simulink model "Quadrotor_Model"  (R2025a)
settings: Solver=ode45  StartTime=0.0  StopTime=370  RelTol=1e-3  EnableMultiTasking=on
values from neighbouring files (symbols this model uses):
  b = 0.07    [project_launch.m]
  drone_mass = 2    [project_launch.m]
  g = 9.81    [project_launch.m]
  Ixx = 0.0231693085    [project_launch.m]
  Iyy = 0.0231693085    [project_launch.m]
  Izz = 0.0449757165    [project_launch.m]
  Jr = 6.8145025e-06    [project_launch.m]
  k = 0.09    [project_launch.m]
  K_d_phi = 0.0002    [project_launch.m]
  K_d_psi = 0.07    [project_launch.m]
  K_d_theta = 0.001    [project_launch.m]
  K_dx = 0.035    [project_launch.m]
  K_dy = 0.06    [project_launch.m]
  K_dz = 5    [project_launch.m]
  K_p_phi = 0.1    [project_launch.m]
  K_p_psi = 0.05    [project_launch.m]
  K_p_theta = 0.75    [project_launch.m]
  K_px = 0.6    [project_launch.m]
  K_py = 0.81    [project_launch.m]
  K_pz = 7    [project_launch.m]
  L = 0.1651    [project_launch.m]
  m = 2    [project_launch.m]
  w = 20    [project_launch.m]
settings Model: Creator=boyan  LastModifiedBy=Happy
settings SolverCC: MaxConsecutiveMinStep=2  AlgebraicLoopSolver=TrustRegion
settings DataIOCC: LimitDataPoints=on  SaveFormat=Array  ReturnWorkspaceOutputs=off
settings OptimizationCC: LifeSpan=inf
settings DebuggingCC: SolverPrmCheckMsg=warning  UnconnectedInputMsg=warning  UnconnectedOutputMsg=warning  UnconnectedLineMsg=warning  SFUnexpectedBacktrackingDiag=warning  SFNoUnconditionalDefaultTransitionDiag=warning  SFExecutionAtInitializationDiag=none  ArithmeticOperatorsInVariantConditions=warning
settings HardwareCC: ProdBitPerPointer=32.0  ProdBitPerSizeT=32.0  ProdBitPerPtrDiffT=32.0  ProdLargestAtomicFloat=None  ProdIntDivRoundTo=Undefined  ProdEndianess=Unspecified  ProdWordSize=32.0  ProdHWDeviceType=32-bit Generic
settings ModelReferenceCC: EnableRefExpFcnMdlSchedulingChecks=on  PropagateSignalLabelsOutOfModel=off
settings SFSimCC: SimUseLocalCustomCode=off  CustomCodeUndefinedFunction=UseInterfaceOnly
settings RTWCC: RTWUseLocalCustomCode=off  GPUComputeCapability=3.5  DLArmComputeVersion=19.05
settings CodeAppCC: StateflowObjectComments=on
settings GRTTargetCC: TargetLangStandard=C89/C90 (ANSI)
settings ConfigComp: CovMetricSettings=dw  CovSaveCumulativeToWorkspaceVar=on  CovSaveSingleToWorkspaceVar=on  CovExternalEMLEnable=off  CovSFcnEnable=off

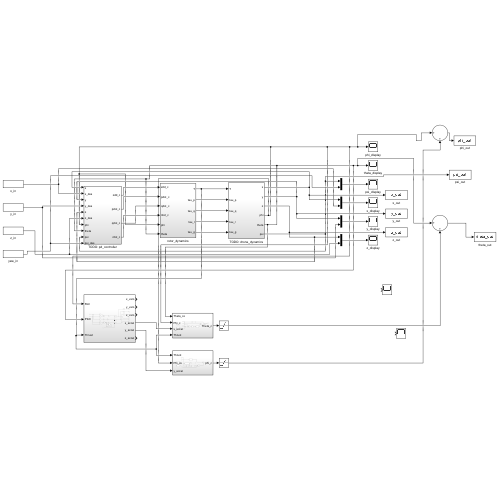
[thumbnail: Simulink's stored preview of the top-level diagram]
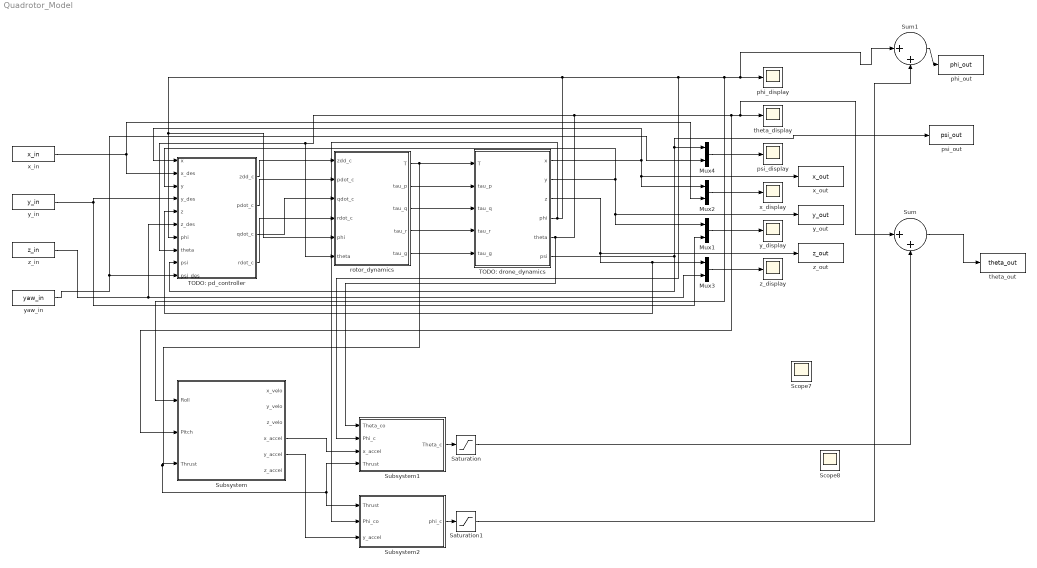
== system Quadrotor_Model ==
  Mux{1..4} (4 alike) : Mux  Inputs=2
  Saturation : Saturate  UpperLimit=160  LowerLimit=-160
  Saturation1 : Saturate  UpperLimit=160  LowerLimit=-160
  Scope7 : Scope
      settings: ActiveDisplayYMinimum=-1.6883197970171271  ActiveDisplayYMaximum=2.5090035346084125  DataLoggingVariableName=ScopeData12
  Scope8 : Scope
      settings: ActiveDisplayYMinimum=-0.67404865904457345  ActiveDisplayYMaximum=1.0700258804030376  DataLoggingVariableName=ScopeData10
  Subsystem : Subsystem
  Subsystem1 : Subsystem
  Subsystem2 : Subsystem
  Sum : Sum  Inputs=|++
  Sum1 : Sum  Inputs=|++
  TODO: drone_dynamics : Subsystem
  TODO: pd_controller : Subsystem
  phi_display : Scope
      settings: ActiveDisplayYMinimum=-3.14  ActiveDisplayYMaximum=3.14
  phi_out : ToWorkspace  VariableName=phi_out  SaveFormat=Timeseries  SampleTime=-1
  psi_display : Scope
      settings: ActiveDisplayYMinimum=-0.78539816339744806  ActiveDisplayYMaximum=7.0685834705770345  DataLoggingVariableName=ScopeData2
  psi_out : ToWorkspace  VariableName=psi_out  SaveFormat=Timeseries  SampleTime=-1
  rotor_dynamics : Subsystem
  theta_display : Scope
      settings: ActiveDisplayYMinimum=-3.14  ActiveDisplayYMaximum=3.14  DataLoggingVariableName=ScopeData3
  theta_out : ToWorkspace  VariableName=theta_out  SaveFormat=Timeseries  SampleTime=-1
  x_display : Scope
      settings: ActiveDisplayYMinimum=-200  DataLoggingVariableName=ScopeData4
  x_in : FromWorkspace  VariableName=x_in
  x_out : ToWorkspace  VariableName=x_out  SaveFormat=Timeseries  SampleTime=-1
  y_display : Scope
      settings: ActiveDisplayYMinimum=-20  ActiveDisplayYMaximum=140  DataLoggingVariableName=ScopeData5
  y_in : FromWorkspace  VariableName=y_in
  y_out : ToWorkspace  VariableName=y_out  SaveFormat=Timeseries  SampleTime=-1
  yaw_in : FromWorkspace  VariableName=yaw_in
  z_display : Scope
      settings: ActiveDisplayYMinimum=-50
  z_in : FromWorkspace  VariableName=z_in
  z_out : ToWorkspace  VariableName=z_out  SaveFormat=Timeseries  SampleTime=-1
  wires:
  rotor_dynamics/2(tau_p) -> TODO: drone_dynamics/2(tau_p)
  TODO: pd_controller/1(zdd_c) -> rotor_dynamics/1(zdd_c)
  TODO: pd_controller/2(pdot_c) -> rotor_dynamics/2(pdot_c)
  z_in/1 -> TODO: pd_controller/6(z_des), Mux3/2
  Mux1/1 -> y_display/1
  Mux2/1 -> x_display/1
  Mux4/1 -> psi_display/1
  Mux3/1 -> z_display/1
  TODO: drone_dynamics/6(psi) -> TODO: pd_controller/9(psi), psi_out/1, Mux4/1
  y_in/1 -> Mux1/2, TODO: pd_controller/4(y_des)
  x_in/1 -> Mux2/2, TODO: pd_controller/2(x_des)
  TODO: drone_dynamics/3(z) -> z_out/1, TODO: pd_controller/5(z), Mux3/1
  TODO: drone_dynamics/5(theta) -> Subsystem1/1(Theta_co), Subsystem/2(Pitch), Sum/1, theta_display/1, rotor_dynamics/6(theta), TODO: pd_controller/8(theta)
  TODO: drone_dynamics/2(y) -> Mux1/1, y_out/1, TODO: pd_controller/3(y)
  TODO: drone_dynamics/4(phi) -> Subsystem2/2(Phi_co), Subsystem1/2(Phi_c), Subsystem/1(Roll), Sum1/1, phi_display/1, rotor_dynamics/5(phi), TODO: pd_controller/7(phi)
  TODO: drone_dynamics/1(x) -> Mux2/1, x_out/1, TODO: pd_controller/1(x)
  rotor_dynamics/5(tau_g) -> TODO: drone_dynamics/5(tau_g)
  rotor_dynamics/3(tau_q) -> TODO: drone_dynamics/3(tau_q)
  rotor_dynamics/4(tau_r) -> TODO: drone_dynamics/4(tau_r)
  yaw_in/1 -> Mux4/2, TODO: pd_controller/10(psi_des)
  TODO: pd_controller/4(rdot_c) -> rotor_dynamics/4(rdot_c)
  TODO: pd_controller/3(qdot_c) -> rotor_dynamics/3(qdot_c)
  rotor_dynamics/1(T) -> Subsystem/3(Thrust), Subsystem1/4(Thrust), Subsystem2/1(Thrust), TODO: drone_dynamics/1(T)
  Saturation1/1 -> Sum1/2
  Subsystem/5(y_accel) -> Subsystem2/3(y_accel)
  Subsystem2/1(phi_c) -> Saturation1/1
  Subsystem1/1(Theta_c) -> Saturation/1
  Subsystem/4(x_accel) -> Subsystem1/3(x_accel)
  Sum/1 -> theta_out/1
  Saturation/1 -> Sum/2
  Sum1/1 -> phi_out/1

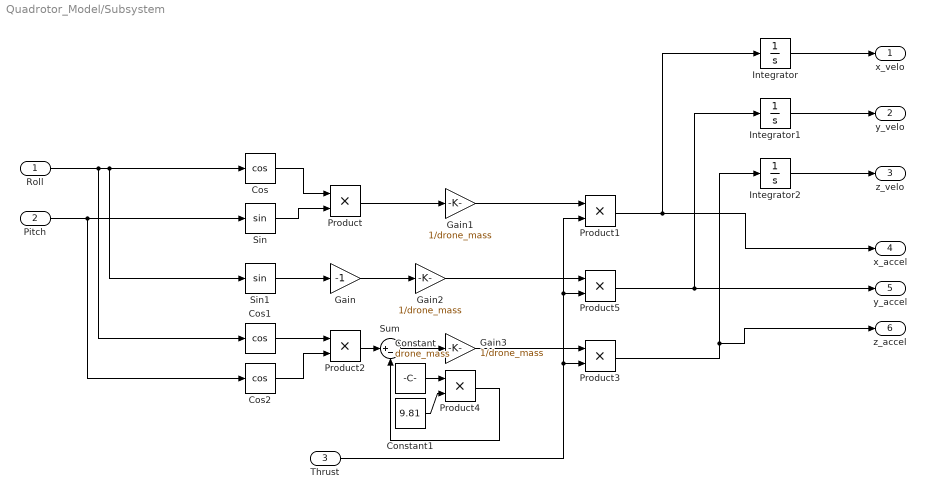
== system Quadrotor_Model/Subsystem ==
  Roll : Inport
  Pitch : Inport  Port=2
  Thrust : Inport  Port=3
  Constant : Constant  Value=drone_mass
  Constant1 : Constant  Value=9.81
  Cos : Trigonometry  Operator=cos
  Cos1 : Trigonometry  Operator=cos
  Cos2 : Trigonometry  Operator=cos
  Gain : Gain  Gain=-1
  Gain1 : Gain  Gain=1/drone_mass
  Gain2 : Gain  Gain=1/drone_mass
  Gain3 : Gain  Gain=1/drone_mass
  Integrator : Integrator
  Integrator1 : Integrator
  Integrator2 : Integrator
  Product{,1..5} (6 alike) : Product
  Sin : Trigonometry
  Sin1 : Trigonometry
  Sum : Sum  Inputs=|+-
  x_velo : Outport
  y_velo : Outport  Port=2
  z_velo : Outport  Port=3
  x_accel : Outport  Port=4
  y_accel : Outport  Port=5
  z_accel : Outport  Port=6
  wires:
  Sin/1 -> Product/2
  Cos/1 -> Product/1
  Pitch/1 -> Sin/1, Cos2/1
  Roll/1 -> Cos1/1, Cos/1, Sin1/1
  Sin1/1 -> Gain/1
  Cos2/1 -> Product2/2
  Cos1/1 -> Product2/1
  Constant/1 -> Product4/1
  Constant1/1 -> Product4/2
  Product4/1 -> Sum/2
  Sum/1 -> Gain3/1
  Thrust/1 -> Product1/2, Product5/2, Product3/2
  Gain/1 -> Gain2/1
  Product/1 -> Gain1/1
  Gain1/1 -> Product1/1
  Gain2/1 -> Product5/1
  Product2/1 -> Sum/1
  Product5/1 -> Integrator1/1, y_accel/1
  Product3/1 -> Integrator2/1, z_accel/1
  Integrator2/1 -> z_velo/1
  Integrator1/1 -> y_velo/1
  Integrator/1 -> x_velo/1
  Product1/1 -> Integrator/1, x_accel/1
  Gain3/1 -> Product3/1

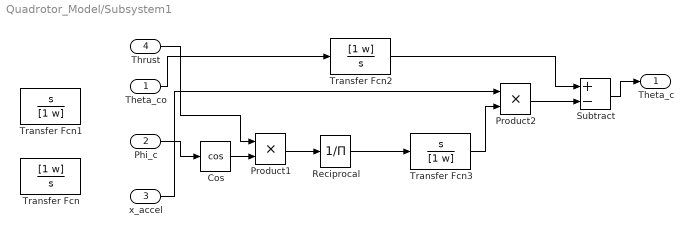
== system Quadrotor_Model/Subsystem1 ==
  Theta_co : Inport
  Phi_c : Inport  Port=2
  x_accel : Inport  Port=3
  Thrust : Inport  Port=4
  Cos : Trigonometry  Operator=cos
  Product1 : Product
  Product2 : Product
  Reciprocal : Product  Inputs=/
  Subtract : Sum  Inputs=+-
  Transfer Fcn : TransferFcn  Numerator=[1 w]  Denominator=[1 0]
  Transfer Fcn1 : TransferFcn  Numerator=[1 0]  Denominator=[1 w]
  Transfer Fcn2 : TransferFcn  Numerator=[1 w]  Denominator=[1 0]
  Transfer Fcn3 : TransferFcn  Numerator=[1 0]  Denominator=[1 w]
  Theta_c : Outport
  wires:
  Theta_co/1 -> Transfer Fcn2/1
  Cos/1 -> Product1/2
  Phi_c/1 -> Cos/1
  Product1/1 -> Reciprocal/1
  x_accel/1 -> Product2/1
  Product2/1 -> Subtract/2
  Transfer Fcn2/1 -> Subtract/1
  Subtract/1 -> Theta_c/1
  Thrust/1 -> Product1/1
  Reciprocal/1 -> Transfer Fcn3/1
  Transfer Fcn3/1 -> Product2/2

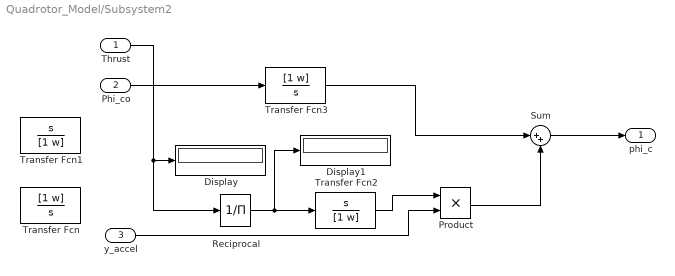
== system Quadrotor_Model/Subsystem2 ==
  Thrust : Inport
  Phi_co : Inport  Port=2
  y_accel : Inport  Port=3
  Display : Display
  Display1 : Display
  Product : Product
  Reciprocal : Product  Inputs=/
  Sum : Sum  Inputs=|++
  Transfer Fcn : TransferFcn  Numerator=[1 w]  Denominator=[1 0]
  Transfer Fcn1 : TransferFcn  Numerator=[1 0]  Denominator=[1 w]
  Transfer Fcn2 : TransferFcn  Numerator=[1 0]  Denominator=[1 w]
  Transfer Fcn3 : TransferFcn  Numerator=[1 w]  Denominator=[1 0]
  phi_c : Outport
  wires:
  Reciprocal/1 -> Display1/1, Transfer Fcn2/1
  y_accel/1 -> Product/2
  Transfer Fcn2/1 -> Product/1
  Product/1 -> Sum/2
  Phi_co/1 -> Transfer Fcn3/1
  Transfer Fcn3/1 -> Sum/1
  Sum/1 -> phi_c/1
  Thrust/1 -> Display/1, Reciprocal/1

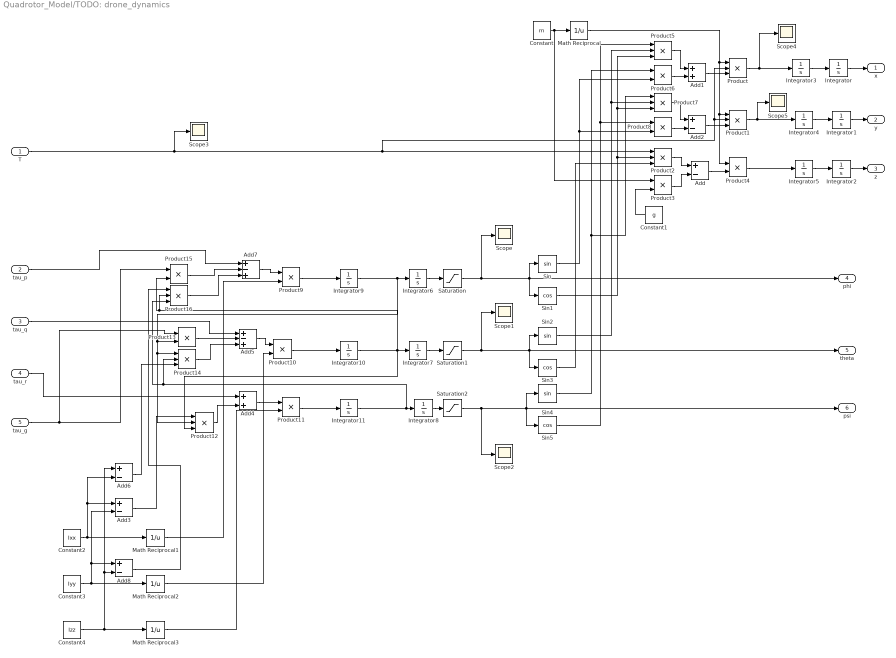
== system Quadrotor_Model/TODO: drone_dynamics ==
  T : Inport
  tau_p : Inport  Port=2
  tau_q : Inport  Port=3
  tau_r : Inport  Port=4
  tau_g : Inport  Port=5
  Add{,2..3,6,8} (5 alike) : Sum  Inputs=+-
  Add1 : Sum
  Add4 : Sum
  Add5 : Sum  Inputs=+-+
  Add7 : Sum  Inputs=+-+
  Constant : Constant  Value=m
  Constant1 : Constant  Value=g
  Constant2 : Constant  Value=Ixx
  Constant3 : Constant  Value=Iyy
  Constant4 : Constant  Value=Izz
  Integrator{,1..7,9..11} (11 alike) : Integrator
  Integrator8 : Integrator  WrappedStateUpperValue=2*pi  WrappedStateLowerValue=0
  Math Reciprocal{,1..3} (4 alike) : Math  Operator=reciprocal  SignedPower=on
  Product{,1..2,5,7,12,14,16} (8 alike) : Product  Inputs=3
  Product{3..4,6,8..11,13,15} (9 alike) : Product
  Saturation : Saturate  UpperLimit=1  LowerLimit=-1
  Saturation1 : Saturate  UpperLimit=1  LowerLimit=-1
  Saturation2 : Saturate  UpperLimit=2*pi  LowerLimit=0
  Scope{,1..5} (6 alike) : Scope
      Scope settings: ActiveDisplayYMinimum=-3.15  ActiveDisplayYMaximum=3.15
      Scope1 settings: ActiveDisplayYMinimum=-4.8E-9  ActiveDisplayYMaximum=6E-10  DataLoggingVariableName=ScopeData2
      Scope2 settings: ActiveDisplayYMinimum=-0.8979  ActiveDisplayYMaximum=7.08108  DataLoggingVariableName=ScopeData3
      Scope3 settings: ActiveDisplayYMinimum=-3.4849041226239738E+14  ActiveDisplayYMaximum=4.4753425626299984E+13  DataLoggingVariableName=ScopeData4
      Scope4 settings: ActiveDisplayYMinimum=-1.5375275296905083E+12  ActiveDisplayYMaximum=8.56477193990877E+11  DataLoggingVariableName=ScopeData5
      Scope5 settings: DataLoggingVariableName=ScopeData6
  Sin : Trigonometry
  Sin1 : Trigonometry  Operator=cos
  Sin2 : Trigonometry
  Sin3 : Trigonometry  Operator=cos
  Sin4 : Trigonometry
  Sin5 : Trigonometry  Operator=cos
  x : Outport
  y : Outport  Port=2
  z : Outport  Port=3
  phi : Outport  Port=4
  theta : Outport  Port=5
  psi : Outport  Port=6
  wires:
  Math Reciprocal1/1 -> Product9/2
  Add5/1 -> Product10/1
  Add7/1 -> Product9/1
  Product9/1 -> Integrator9/1
  Add/1 -> Product4/2
  Product4/1 -> Integrator5/1
  Sin1/1 -> Product2/2, Product7/3, Product5/3
  Constant2/1 -> Math Reciprocal1/1, Add6/2, Add3/1
  Integrator11/1 -> Product16/3, Product14/2, Integrator8/1
  Integrator/1 -> x/1
  Sin/1 -> Product8/2, Product6/2
  Sin3/1 -> Product2/3
  T/1 -> Scope3/1, Product/2, Product1/2, Product2/1
  Constant4/1 -> Math Reciprocal3/1, Add8/2, Add6/1
  Add6/1 -> Product14/3
  Integrator4/1 -> Integrator1/1
  Product5/1 -> Add1/1
  Math Reciprocal3/1 -> Product11/2
  Product11/1 -> Integrator11/1
  Integrator6/1 -> Saturation/1
  Integrator9/1 -> Product12/2, Product14/1, Product13/2, Integrator6/1
  Product6/1 -> Add1/2
  Product14/1 -> Add5/3
  Add8/1 -> Product16/1
  Integrator5/1 -> Integrator2/1
  Constant1/1 -> Product3/2
  Product16/1 -> Add7/3
  Saturation2/1 -> psi/1, Sin5/1, Sin4/1, Scope2/1
  Add1/1 -> Product/3
  Integrator3/1 -> Integrator/1
  Saturation/1 -> phi/1, Sin1/1, Sin/1, Scope/1
  Integrator7/1 -> Saturation1/1
  Sin5/1 -> Product8/1, Product5/1
  tau_p/1 -> Add7/1
  Sin4/1 -> Product7/1, Product6/1
  Constant3/1 -> Add8/1, Add3/2, Math Reciprocal2/1
  Add3/1 -> Product12/1
  Product7/1 -> Add2/1
  Math Reciprocal2/1 -> Product10/2
  Product13/1 -> Add5/2
  Integrator1/1 -> y/1
  Product2/1 -> Add/1
  Add2/1 -> Product1/3
  Product15/1 -> Add7/2
  tau_g/1 -> Product15/1, Product13/1
  Product10/1 -> Integrator10/1
  Sin2/1 -> Product5/2, Product7/2
  Product/1 -> Scope4/1, Integrator3/1
  Product8/1 -> Add2/2
  Math Reciprocal/1 -> Product/1, Product4/1, Product1/1
  Integrator2/1 -> z/1
  Product12/1 -> Add4/2
  Product3/1 -> Add/2
  tau_r/1 -> Add4/1
  Product1/1 -> Scope5/1, Integrator4/1
  Constant/1 -> Math Reciprocal/1, Product3/1
  Saturation1/1 -> Sin3/1, theta/1, Sin2/1, Scope1/1
  Add4/1 -> Product11/1
  Integrator8/1 -> Saturation2/1
  Integrator10/1 -> Product12/3, Product16/2, Product15/2, Integrator7/1
  tau_q/1 -> Add5/1

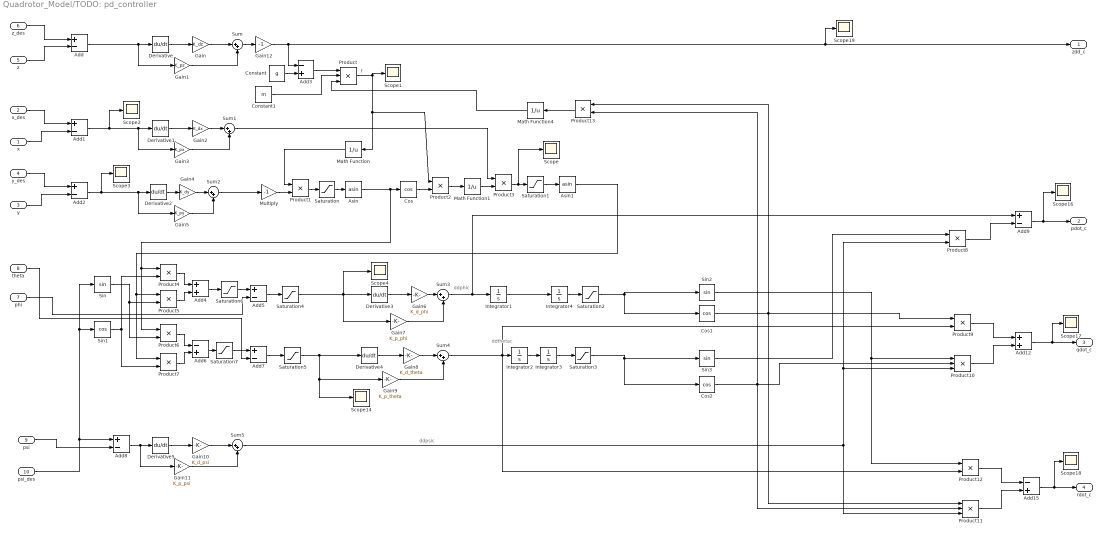
== system Quadrotor_Model/TODO: pd_controller ==
  note: ddphic
  note: ddthetac
  note: f
  note: ddpsic
  x : Inport
  x_des : Inport  Port=2
  y : Inport  Port=3
  y_des : Inport  Port=4
  z : Inport  Port=5
  z_des : Inport  Port=6
  phi : Inport  Port=7
  theta : Inport  Port=8
  psi : Inport  Port=9
  psi_des : Inport  Port=10
  Add{,1..2,5,7..9} (7 alike) : Sum  Inputs=+-
  Add12 : Sum
  Add15 : Sum  Inputs=-+
  Add3 : Sum  Inputs=-+
  Add4 : Sum
  Add6 : Sum  Inputs=-+
  Asin : Trigonometry  Operator=asin
  Asin1 : Trigonometry  Operator=asin
  Constant : Constant  Value=g
  Constant1 : Constant  Value=m
  Cos : Trigonometry  Operator=cos
  Cos1 : Trigonometry  Operator=cos
  Cos2 : Trigonometry  Operator=cos
  Derivative{,1..5} (6 alike) : Derivative
  Gain : Gain  Gain=K_dz
  Gain1 : Gain  Gain=K_pz
  Gain10 : Gain  Gain=K_d_psi
  Gain11 : Gain  Gain=K_p_psi
  Gain12 : Gain  Gain=-1
  Gain2 : Gain  Gain=K_dx
  Gain3 : Gain  Gain=K_px
  Gain4 : Gain  Gain=K_dy
  Gain5 : Gain  Gain=K_py
  Gain6 : Gain  Gain=K_d_phi
  Gain7 : Gain  Gain=K_p_phi
  Gain8 : Gain  Gain=K_d_theta
  Gain9 : Gain  Gain=K_p_theta
  Integrator{1..4} (4 alike) : Integrator
  Math Function : Math  Operator=reciprocal
  Math Function1 : Math  Operator=reciprocal
  Math Function4 : Math  Operator=reciprocal
  Multiply : Gain  Gain=-1
  Product : Product  Inputs=3
  Product{1..9,12..13} (11 alike) : Product
  Product10 : Product  Inputs=3
  Product11 : Product  Inputs=3
  Saturation{,1..3,6..7} (6 alike) : Saturate  UpperLimit=1  LowerLimit=-1  ZeroCross=off
  Saturation4 : Saturate  UpperLimit=0.2  LowerLimit=-0.2  ZeroCross=off
  Saturation5 : Saturate  UpperLimit=0.1  LowerLimit=-0.1  ZeroCross=off
  Scope{,1..4,14,16..19} (10 alike) : Scope
      Scope settings: ActiveDisplayYMinimum=-3E-11  ActiveDisplayYMaximum=2E-10  DataLoggingVariableName=ScopeData7
      Scope1 settings: ActiveDisplayYMinimum=-4.3522364874412031E+14  ActiveDisplayYMaximum=5.24366948093118E+13
      Scope14 settings: ActiveDisplayYMinimum=-2.2  ActiveDisplayYMaximum=2.2  DataLoggingVariableName=ScopeData13
      Scope16 settings: ActiveDisplayYMinimum=-0.00891  ActiveDisplayYMaximum=0.00408  DataLoggingVariableName=ScopeData15
      Scope17 settings: ActiveDisplayYMinimum=-0.01  ActiveDisplayYMaximum=0.01  DataLoggingVariableName=ScopeData16
      Scope18 settings: ActiveDisplayYMinimum=-1.1  ActiveDisplayYMaximum=1.1  DataLoggingVariableName=ScopeData17
      Scope19 settings: ActiveDisplayYMinimum=-3.30547176345424E+9  ActiveDisplayYMaximum=2.2541333614408321E+10  DataLoggingVariableName=ScopeData18
      Scope2 settings: ActiveDisplayYMinimum=-15  ActiveDisplayYMaximum=15  DataLoggingVariableName=ScopeData2
      Scope3 settings: DataLoggingVariableName=ScopeData3
      Scope4 settings: ActiveDisplayYMinimum=-0.25  ActiveDisplayYMaximum=0.25  DataLoggingVariableName=ScopeData4
  Sin : Trigonometry
  Sin1 : Trigonometry  Operator=cos
  Sin2 : Trigonometry
  Sin3 : Trigonometry
  Sum{,1..5} (6 alike) : Sum  Inputs=|++
  zdd_c : Outport
  pdot_c : Outport  Port=2
  qdot_c : Outport  Port=3
  rdot_c : Outport  Port=4
  wires:
  Cos2/1 -> Product13/2, Product11/2, Product10/2
  Derivative4/1 -> Gain8/1
  Math Function1/1 -> Product3/2
  Gain11/1 -> Sum5/2
  psi_des/1 -> Add8/1, Sin/1, Sin1/1
  Multiply/1 -> Product1/2
  Math Function4/1 -> Product/3
  Gain9/1 -> Sum4/2
  Derivative5/1 -> Gain10/1
  theta/1 -> Add7/2
  Gain5/1 -> Sum2/2
  Add6/1 -> Saturation7/1
  Saturation2/1 -> Cos1/1, Sin2/1
  Product6/1 -> Add6/1
  Gain4/1 -> Sum2/1
  Integrator2/1 -> Integrator3/1
  Sum3/1 -> Add9/1, Integrator1/1
  Derivative/1 -> Gain/1
  Add/1 -> Gain1/1, Derivative/1
  Sin/1 -> Product6/2, Product5/2
  Gain7/1 -> Sum3/2
  Add2/1 -> Scope3/1, Gain5/1, Derivative2/1
  Product13/1 -> Math Function4/1
  Product11/1 -> Add15/2
  x_des/1 -> Add1/1
  Product4/1 -> Add4/1
  Add15/1 -> rdot_c/1, Scope18/1
  Asin1/1 -> Product7/1, Product5/1
  Sum5/1 -> Product11/3, Product10/3, Product8/2
  Product8/1 -> Add9/2
  Derivative2/1 -> Gain4/1
  Gain1/1 -> Sum/2
  Asin/1 -> Product4/1, Product6/1, Cos/1
  Sum2/1 -> Multiply/1
  Gain8/1 -> Sum4/1
  Constant1/1 -> Product/2
  Add1/1 -> Scope2/1, Gain3/1, Derivative1/1
  Derivative3/1 -> Gain6/1
  Product9/1 -> Add12/1
  Math Function/1 -> Product1/1
  Gain3/1 -> Sum1/2
  x/1 -> Add1/2
  Product5/1 -> Add4/2
  Cos/1 -> Product2/2
  Sin1/1 -> Product7/2, Product4/2
  Sum/1 -> Gain12/1
  Integrator1/1 -> Integrator4/1
  Add12/1 -> qdot_c/1, Scope17/1
  Integrator3/1 -> Saturation3/1
  Product1/1 -> Saturation/1
  Integrator4/1 -> Saturation2/1
  Gain/1 -> Sum/1
  Add3/1 -> Product/1
  Saturation1/1 -> Asin1/1
  Sum4/1 -> Product12/2, Product9/2, Integrator2/1
  Sin3/1 -> Product8/1
  Product2/1 -> Math Function1/1
  Gain2/1 -> Sum1/1
  z_des/1 -> Add/1
  Cos1/1 -> Product13/1, Product11/1, Product9/1
  Gain10/1 -> Sum5/1
  Constant/1 -> Add3/2
  Add9/1 -> pdot_c/1, Scope16/1
  Sum1/1 -> Product3/1
  Product3/1 -> Scope/1, Saturation1/1
  Add8/1 -> Derivative5/1, Gain11/1
  Product10/1 -> Add12/2
  Product12/1 -> Add15/1
  y/1 -> Add2/2
  Add4/1 -> Saturation6/1
  Derivative1/1 -> Gain2/1
  Gain6/1 -> Sum3/1
  Sin2/1 -> Product12/1, Product10/1
  Product7/1 -> Add6/2
  y_des/1 -> Add2/1
  Product/1 -> Product2/1, Math Function/1, Scope1/1
  z/1 -> Add/2
  Saturation3/1 -> Cos2/1, Sin3/1
  psi/1 -> Add8/2
  Saturation/1 -> Asin/1
  phi/1 -> Add5/2
  Gain12/1 -> zdd_c/1, Scope19/1, Add3/1
  Saturation6/1 -> Add5/1
  Add5/1 -> Saturation4/1
  Saturation7/1 -> Add7/1
  Add7/1 -> Saturation5/1
  Saturation4/1 -> Derivative3/1, Scope4/1, Gain7/1
  Saturation5/1 -> Scope14/1, Gain9/1, Derivative4/1

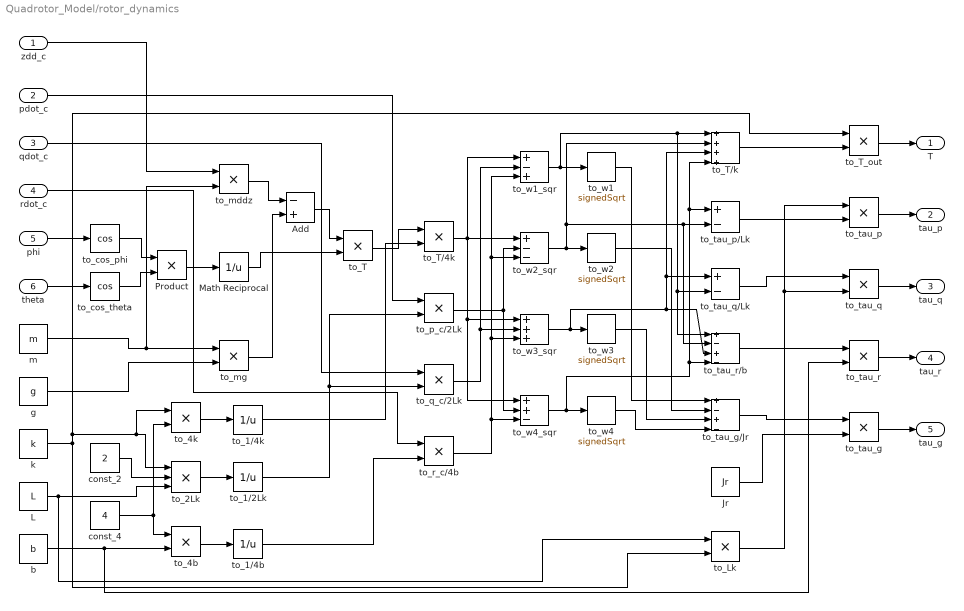
== system Quadrotor_Model/rotor_dynamics ==
  zdd_c : Inport
  pdot_c : Inport  Port=2
  qdot_c : Inport  Port=3
  rdot_c : Inport  Port=4
  phi : Inport  Port=5
  theta : Inport  Port=6
  Add : Sum  Inputs=-+
  Jr : Constant  Value=Jr
  L : Constant  Value=L
  Math Reciprocal : Math  Operator=reciprocal  SignedPower=on
  Product : Product
  b : Constant  Value=b
  const_2 : Constant  Value=2
  const_4 : Constant  Value=4
  g : Constant  Value=g
  k : Constant  Value=k
  m : Constant  Value=m
  to_1/2Lk : Math  Operator=reciprocal  SignedPower=on
  to_1/4b : Math  Operator=reciprocal  SignedPower=on
  to_1/4k : Math  Operator=reciprocal  SignedPower=on
  to_2Lk : Product  Inputs=3
  to_4b : Product
  to_4k : Product
  to_Lk : Product
  to_T : Product
  to_T/4k : Product
  to_T/k : Sum  Inputs=++++
  to_T_out : Product
  to_cos_phi : Trigonometry  Operator=cos
  to_cos_theta : Trigonometry  Operator=cos
  to_mddz : Product
  to_mg : Product
  to_p_c/2Lk : Product
  to_q_c/2Lk : Product
  to_r_c/4b : Product
  to_tau_g : Product
  to_tau_g/Jr : Sum  Inputs=+-+-
  to_tau_p : Product
  to_tau_p/Lk : Sum  Inputs=+-
  to_tau_q : Product
  to_tau_q/Lk : Sum  Inputs=+-
  to_tau_r : Product
  to_tau_r/b : Sum  Inputs=+-+-
  to_w{1..4} (4 alike) : Sqrt  Operator=signedSqrt
  to_w1_sqr : Sum  Inputs=+-+
  to_w2_sqr : Sum  Inputs=+--
  to_w3_sqr : Sum  Inputs=+++
  to_w4_sqr : Sum  Inputs=++-
  T : Outport
  tau_p : Outport  Port=2
  tau_q : Outport  Port=3
  tau_r : Outport  Port=4
  tau_g : Outport  Port=5
  wires:
  phi/1 -> to_cos_phi/1
  theta/1 -> to_cos_theta/1
  to_cos_phi/1 -> Product/1
  to_cos_theta/1 -> Product/2
  Product/1 -> Math Reciprocal/1
  m/1 -> to_mddz/2, to_mg/1
  g/1 -> to_mg/2
  to_mg/1 -> Add/2
  Math Reciprocal/1 -> to_T/2
  Add/1 -> to_T/1
  k/1 -> to_2Lk/1, to_4k/1, to_T_out/1, to_Lk/2
  const_4/1 -> to_4b/1, to_4k/2
  const_2/1 -> to_2Lk/2
  L/1 -> to_2Lk/3, to_Lk/1
  b/1 -> to_tau_r/2, to_4b/2
  to_4k/1 -> to_1/4k/1
  to_2Lk/1 -> to_1/2Lk/1
  to_4b/1 -> to_1/4b/1
  to_T/1 -> to_T/4k/1
  to_1/4k/1 -> to_T/4k/2
  pdot_c/1 -> to_p_c/2Lk/1
  to_1/2Lk/1 -> to_q_c/2Lk/2, to_p_c/2Lk/2
  qdot_c/1 -> to_q_c/2Lk/1
  to_1/4b/1 -> to_r_c/4b/2
  rdot_c/1 -> to_r_c/4b/1
  to_T/4k/1 -> to_w2_sqr/1, to_w3_sqr/1, to_w4_sqr/1, to_w1_sqr/1
  to_q_c/2Lk/1 -> to_w3_sqr/2, to_w1_sqr/2
  to_r_c/4b/1 -> to_w4_sqr/3, to_w3_sqr/3, to_w2_sqr/3, to_w1_sqr/3
  to_p_c/2Lk/1 -> to_w2_sqr/2, to_w4_sqr/2
  to_w1_sqr/1 -> to_w1/1, to_tau_r/b/1, to_tau_q/Lk/2, to_T/k/1
  to_w2_sqr/1 -> to_w2/1, to_tau_r/b/2, to_tau_p/Lk/2, to_T/k/2
  to_w3_sqr/1 -> to_w3/1, to_tau_q/Lk/1, to_T/k/3, to_tau_r/b/3
  to_w4_sqr/1 -> to_w4/1, to_tau_p/Lk/1, to_T/k/4, to_tau_r/b/4
  to_w2/1 -> to_tau_g/Jr/2
  to_w1/1 -> to_tau_g/Jr/1
  to_w3/1 -> to_tau_g/Jr/3
  to_w4/1 -> to_tau_g/Jr/4
  to_T_out/1 -> T/1
  to_T/k/1 -> to_T_out/2
  to_tau_p/1 -> tau_p/1
  to_tau_p/Lk/1 -> to_tau_p/2
  to_tau_q/1 -> tau_q/1
  to_tau_r/1 -> tau_r/1
  to_tau_r/b/1 -> to_tau_r/1
  to_tau_q/Lk/1 -> to_tau_q/1
  to_tau_g/1 -> tau_g/1
  to_tau_g/Jr/1 -> to_tau_g/1
  to_Lk/1 -> to_tau_p/1, to_tau_q/2
  Jr/1 -> to_tau_g/2
  zdd_c/1 -> to_mddz/1
  to_mddz/1 -> Add/1
